simulink model "system2020b"  (R2020b)
settings: Solver=VariableStepAuto  StartTime=0.0  StopTime=50  RelTol=1e-3
InitFcn:
  | parametriEgo
values from neighbouring files (symbols this model uses):
  campnormalized = campmag/sqrt(campmag(1)^2+campmag(2)^2+campmag(3)^2)    [parametriEgo.m]
  g = 9.81    [kalman_jacobian.m]    (also in parametriEgo.m = [0; 0; -9.81])
  initial_conditions = [0,0,0*pi/180,0*pi/180,0,0]    [parametriEgo.m]
  k_e_qf = 0.1    [ego_control_gains_sensors.m]
  ki_e_nu_speed = 2.5    [ego_control_gains_sensors.m]
  kp_e_nu_phidot = 7    [ego_control_gains_sensors.m]
  kp_e_nu_speed = 6    [ego_control_gains_sensors.m]
  kp_e_nu_thetadot = 7    [ego_control_gains_sensors.m]
  kp_e_theta = 40    [ego_control_gains_sensors.m]
  l = 0.248    [parametriEgo.m]
  L = 0.379    [parametriEgo.m]
  mb = 21.7+0.536*10+0.381*2    (= 27.822)    [parametriEgo.m]
  mw = 1.6    [parametriEgo.m]
  P0 = 1500*eye(7)    [parametriEgo.m]
  r = 0.13    [parametriEgo.m]
  seedAcc1 = ceil(rand()*10)    [parametriEgo.m]
  seedAcc2 = ceil(rand()*10)    [parametriEgo.m]
  seedGyro1 = ceil(rand()*10)    [parametriEgo.m]
  seedGyro2 = ceil(rand()*10)    [parametriEgo.m]
  tau_max = 11    [parametriEgo.m]
  totAccNoisePower = (accNoiseDens* 10^-6 * 9.8)^2    (= 8.6436e-06)    [parametriEgo.m]
  totGyroNoisePower = (gyroNoiseDens * pi/180)^2    (= 3.04617419787e-06)    [parametriEgo.m]
  Ts = 1/100    (= 0.01)    [parametriEgo.m]
  TsController = 1/100    (= 0.01)    [parametriEgo.m]
  TsGraph = 1/100    (= 0.01)    [parametriEgo.m]
  x0 = zeros(7,1)    [parametriEgo.m]
undefined symbols (not defined in the file or in its folder): alpha
libraries: simulink_extras x45, simulink x10, eeGeneralControl x3
(part 3 of 3)

== matlab function system2020b/Physical system/old model/LQR con linearizzato/LQR ==
  data: A_ss input; K output; B_ss input
function K = fcn(A_ss, B_ss)

Q = eye(6);
R = eye(2);

% state: nu1, nu2, nu3, nu1_int, theta, phi

Q = [500,0,0,0,0,0;
    0,10,0,0,0,0;
    0,0,10,0,0,0;
    0,0,0,10000,0,0;
    0,0,0,0,100,0;
    0,0,0,0,0,400];

R = [0.1,0;
    0,0.1];

coder.extrinsic('lqr')

K = zeros(2, 6);

K = lqr(A_ss, B_ss, Q, R);
end

== matlab function system2020b/Sensors/accelerometer/rotation matrix I->B ==
  data: u input; y output
function y = fcn(u)
% Robotics project, Menolotto Mariangela & Stefano Maugeri

theta = u(3);
phi = u(4);

%Ralpha = [1, 0, 0; 0, cos(alpha), -sin(alpha); 0, sin(alpha), cos(alpha)];
Rtheta = [cos(theta), -sin(theta), 0; sin(theta), cos(theta), 0; 0, 0, 1];
Rphi = [1, 0, 0; 0, cos(phi), -sin(phi); 0, sin(phi), cos(phi)];

y = Rphi'*Rtheta';

== matlab function system2020b/Sensors/accelerometer/rotation matrix1 ==
  data: u input; alpha input; y output
function y=fcn(u, alpha)
% Robotics project, Menolotto Mariangela & Stefano Maugeri

theta = u(3);
phi = u(4);

Ralpha = [1, 0, 0; 0, cos(alpha), -sin(alpha); 0, sin(alpha), cos(alpha)];
Rtheta = [cos(theta), -sin(theta), 0; sin(theta), cos(theta), 0; 0, 0, 1];
Rphi = [1, 0, 0; 0, cos(phi), -sin(phi); 0, sin(phi), cos(phi)];

y = Rphi'*Rtheta' * Ralpha';

== matlab function system2020b/Filtering/Mahony + distance sensor/mahony filter/MATLAB Function ==
  data: acc input; R output; gyro input; mb input; Rprev input; I output; Iprev input; Ts parameter; campnormalized parameter
function [R, I] = fcn(acc, gyro, mb, Rprev, Iprev, Ts, campnormalized)
% Robotics project, Menolotto Mariangela & Stefano Maugeri

dt = Ts;

%kp=4; oppure 6
%ki=1.2;
% kp=3.5;
% ki=1.3;
kp=1.5; % 1.5
ki=0;
l_acc = 1; 
l_mag = 0.5;


mod_a = sqrt(acc(1)^2+acc(2)^2+acc(3)^2);

acc = acc/mod_a;
mb = mb/norm(mb);

e_a = cross(acc, Rprev'*[0,0,1]'); % g è normalizzato
e_m = cross(mb, Rprev'*campnormalized');

e = l_acc * e_a + l_mag * e_m;

%I = Iprev+ki*e/dt;
I = Iprev+ki*e*dt;

deomega = kp*e + I;
    
omega = deomega + gyro;

omegaSkew = [0, - omega(3), omega(2); omega(3), 0, -omega(1); -omega(2), omega(1), 0];

Re = Rprev + Rprev * omegaSkew * dt;

[U, D, V] = svd(Re);

sigma = det(U*V');

R = U * diag([1,1,sigma]) * V';

== matlab function system2020b/Filtering/Kalman filter/EKF ==
  data: theta_wheels input; acc input; theta_dot output; gyro input; magn input; x input; P input; phi_dot output; angles output; x output; P output; Ts parameter; l parameter; r parameter
% Robotics project, Menolotto Mariangela & Stefano Maugeri
function [theta_dot, phi_dot, angles, x, P] = fcn(theta_wheels, acc, gyro, magn, x, P, Ts, l, r)
%
%           alpha
%           theta
%           phi
% state x = theta dot
%           phi dot
%           x dot dot
%           y dot dot
%
%% init
angles = zeros(3,1);
g = 9.81;
m_e = [0.238836 -0.010851 0.392423];
y=zeros(9,1);
y_err=zeros(9,1);
H = zeros(9,7);
theta_old = x(2);
gamma = 0.05;
beta = 0;
%% Pesi
%R = diag([50,50,50,200,200,200,250,250,250]);
% ultima R=diag([ 50*ones(1,3), 80*ones(1,3), 250*ones(1,3)]);
R=diag([ 0.01*ones(1,3), 0.01*ones(1,3), 0.01*ones(1,3)]);

% gyro1, gyro2, gyro3, acc1, acc2, acc3, mag1, mag2, mag3

%Q = diag([0.0005, 0.00005, 0.000001, 5, 5, 500000, 500000])/20;
Q = diag([0.0005, 0.000001, 0.000001, 5, 5, 500000, 500000])/20;

% alpha, theta, phi, theta dot, phi dot, x dot dot, y dot dot

%%
mx=m_e(1);
my=m_e(2);
mz=m_e(3);

y(1) = gyro(1);
y(2) = gyro(2);
y(3) = gyro(3);
y(4) = acc(1);
y(5) = acc(2);
y(6) = acc(3);
y(7) = magn(1);
y(8) = magn(2);
y(9) = magn(3);


%%

y_err(1) = y(1) - x(5);
y_err(2) = y(2) - sin(x(3))*x(4);
y_err(3) = y(3) - cos(x(3))*x(4);
y_err(4) = y(4) - (sin(x(1))*sin(x(2))*g + cos(x(2))*x(6) + sin(x(2))*x(7));
y_err(5) = y(5) - ((cos(x(2))*cos(x(3))*sin(x(1)) + cos(x(1))*sin(x(3)))*g - cos(x(3))*sin(x(2))*x(6) + cos(x(2))*cos(x(3))*x(7));
y_err(6) = y(6) - ((cos(x(1))*cos(x(3)) - sin(x(1))*cos(x(2))*sin(x(3)) )*g + sin(x(3))*sin(x(2))*x(6) - cos(x(2))*sin(x(3))*x(7));
y_err(7) = y(7) - (mx*cos(x(2)) + (my*cos(x(1))+mz*sin(x(1)))*sin(x(2)));
y_err(8) = y(8) - (mz*cos(x(2))*cos(x(3))*sin(x(1)) - mx*cos(x(3))*sin(x(2)) - my*sin(x(1))*sin(x(3)) + cos(x(1))*( my*cos(x(2))*cos(x(3)) + mz*sin(x(3)) )   );
y_err(9) = y(9) - ( cos(x(3))* (mz*cos(x(1)) - my*sin(x(1))) - cos(x(2))*(my*cos(x(1))+mz*sin(x(1)))*sin(x(3))+ mx*sin(x(2))*sin(x(3)) );

% H = kalman_jacobian

%%

%           alpha
%           theta
%           phi
% state x = theta dot
%           phi dot
%           x dot dot
%           y dot dot

alpha = x(1);
theta = x(2);
phi = x(3);
phidot=x(4);
thetadot=x(5);
xdotdot=x(6);
ydotdot=x(7);

H = Hkalman(alpha,phi,theta,thetadot,xdotdot,ydotdot);

% H = (9,7)
% P = (7,7)
% R = (9,9)
% K = (7,9)
% x = (7,1)
% S = (9,9)

%% predizione
% x = x;
% x(2) = x(2) + x(4) * Ts;
% % x(2) = r/(2*l) *(theta_wheels(2)-theta_wheels(1));
% x(3) = (x(3) + x(5) * Ts)*(1-beta) + x(3)*beta;
% x(4) = ((x(2)-theta_old)/Ts)*gamma + x(4)*(1-gamma);

x(2) = x(2) + x(4) * Ts;
x(3) = x(3) + x(5) * Ts;

F = eye(7);

F(2,4)=Ts;
F(3,5)=Ts;

P = F*P*F' + Q;


%% correzione
S = H * P * H' + R;
K = P * H' * inv(S);
x = x + K*y_err;
P = (eye(7) - K*H) * P;

%% 
angles(1) = x(1);
angles(2) = x(2);
angles(3) = x(3);
theta_dot = x(4);
phi_dot = x(5);
